simulink model "fixpt_acc_data"  (R2015b)
settings: Solver=FixedStepDiscrete  SolverMode=SingleTasking  StartTime=0.0  StopTime=10  RelTol=1e-3
settings Model: DataTypeOverride=Off  Creator=amatsumo  LastModifiedBy=amatsumo
settings DataIOCC: SaveFormat=Array  SaveOutput=off  SignalLogging=off  SaveTime=off
settings OptimizationCC: BlockReduction=off  ConditionallyExecuteInputs=off  DefaultParameterBehavior=Inlined
settings DebuggingCC: AlgebraicLoopMsg=error  UnderspecifiedInitializationDetection=Classic  MergeDetectMultiDrivingBlocksExec=none  SolverPrmCheckMsg=warning  InheritedTsInSrcMsg=none  SingleTaskRateTransMsg=error  StateNameClashWarn=warning
settings HardwareCC: ProdBitPerPointer=32  ProdLargestAtomicFloat=None  ProdIntDivRoundTo=Undefined  ProdEndianess=Unspecified  ProdWordSize=32  ProdHWDeviceType=ASIC/FPGA->ASIC/FPGA  ProdEqTarget=off
settings GRTTargetCC: GeneratePreprocessorConditionals=Disable all
settings ConfigComp: CovModelRefEnable=Off  CovSFcnEnable=off

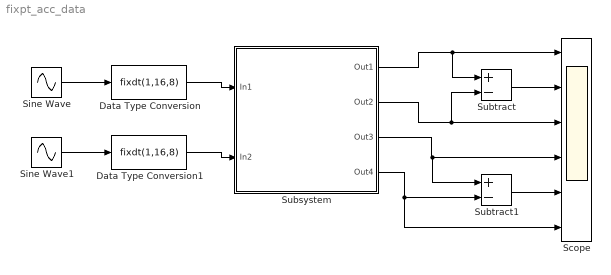
== system fixpt_acc_data ==
  Data Type Conversion : DataTypeConversion  OutDataTypeStr=fixdt(1,16,8)
  Data Type Conversion1 : DataTypeConversion  OutDataTypeStr=fixdt(1,16,8)
  Scope : Scope  NumInputPorts=6
  Sine Wave : Sin  Frequency=2*pi  SampleTime=1/100
  Sine Wave1 : Sin  Frequency=2*pi*2.8  SampleTime=1/100
  Subsystem : Subsystem
  Subtract : Sum  Inputs=+-
  Subtract1 : Sum  Inputs=+-
  wires:
  Sine Wave/1 -> Data Type Conversion/1
  Sine Wave1/1 -> Data Type Conversion1/1
  Subtract/1 -> Scope/2
  Data Type Conversion/1 -> Subsystem/1(In1)
  Data Type Conversion1/1 -> Subsystem/2(In2)
  Subsystem/1(Out1) -> Subtract/1, Scope/1
  Subsystem/2(Out2) -> Subtract/2, Scope/3
  Subtract1/1 -> Scope/5
  Subsystem/3(Out3) -> Subtract1/1, Scope/4
  Subsystem/4(Out4) -> Scope/6, Subtract1/2

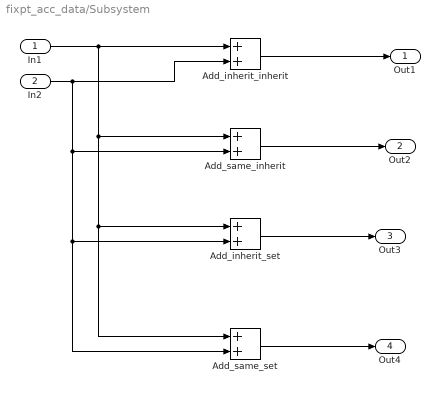
== system fixpt_acc_data/Subsystem ==
  In1 : Inport
  In2 : Inport  Port=2
  Add_inherit_inherit : Sum
      settings: AttributesFormatString=%<AccumDataTypeStr>\n%<OutDataTypeStr>
  Add_inherit_set : Sum  OutDataTypeStr=fixdt(1,14,7)
      settings: AttributesFormatString=%<AccumDataTypeStr>\n%<OutDataTypeStr>
  Add_same_inherit : Sum
      settings: AttributesFormatString=%<AccumDataTypeStr>\n%<OutDataTypeStr>
  Add_same_set : Sum  OutDataTypeStr=fixdt(1,14,7)
      settings: AttributesFormatString=%<AccumDataTypeStr>\n%<OutDataTypeStr>
  Out1 : Outport
  Out2 : Outport  Port=2
  Out3 : Outport  Port=3
  Out4 : Outport  Port=4
  wires:
  In2/1 -> Add_same_set/2, Add_inherit_set/2, Add_same_inherit/2, Add_inherit_inherit/2
  In1/1 -> Add_same_inherit/1, Add_same_set/1, Add_inherit_set/1, Add_inherit_inherit/1
  Add_inherit_inherit/1 -> Out1/1
  Add_inherit_set/1 -> Out3/1
  Add_same_inherit/1 -> Out2/1
  Add_same_set/1 -> Out4/1
